simulink model "uvms_sliding_quaternions"  (Simulink 7.9)
settings: Solver=ode4  StartTime=0.0  StopTime=10  FixedStep=dt  RelTol=2*1e-3
values from neighbouring files (symbols this model uses):
  DH = struct('a',zeros(n,1),'d',zeros(n,1),'alpha',zeros(n,1))    [init.m]
  dt = read_config('dt', 'number')    [run_simulation.m]
undefined symbols (not defined in the file or in its folder): commanded_zeta, ee_pose_init, ee_pose_quaternion_init, Kinetics_Parameters, q_init, V_current, vehicle_position_init, vehicle_quaternion_init
libraries: simulink x1
(part 2 of 2)

== matlab function Controller/sliding mode 2/tau1 ==
  data: Kinetics_Parameters input Bus: kinetics_bus; tau output double; Measured_States input Bus: measured_states_bus; Commanded_States input Bus: commanded_states_bus; zetas input double; dzetas input double
function tau = slidingMode(Kinetics_Parameters, Measured_States,Commanded_States, zetas, dzetas)
%#codegen
    
    
    zeta = Measured_States.zeta;
    zetar_est = zeta;
    s = zeta - zetas;
    Mest = 0.9*getM(Measured_States, Kinetics_Parameters);
    Cest = 1.2*getC(Measured_States, Kinetics_Parameters, zeta, zetar_est);
    Dest = 1.3*getD(Measured_States, Kinetics_Parameters, zetar_est);
    Nest = 0.75*getN(Measured_States, Kinetics_Parameters);
    Xiest = zeros(12,1);

    Kd=diag([10, 10, 10 ,15, 20, 15, ...
             10, 10, 10, 10, 10, 10])*1.2;
    Ks=diag([50, 50, 50, 60, 80, 60, ...
             10, 10, 10, 10, 10, 10])*1.5;
   
    tau = Mest* dzetas + Cest* zetas + Dest * zetas + Nest + Xiest - Kd* s - Ks*sat( s, 0.3) ;% Ks*sat( s, 0.5);
    
end

%------------------------------------------------------------------------
% saturation function
function vec = sat (x,epsilon)
    vec=zeros(length(x),1);
    for i=1:length(x)
       if x(i) > epsilon
           vec(i)=1;
       elseif x(i) < -epsilon
           vec(i)=-1;
       else
           vec(i)=x(i)/epsilon;
       end
    end
end


%% --------------------------------------------------------------
%  Functions to gather the vectors   
%%---------------------------------------------------------------

function M = getM(Measured_States, Kinetics_Parameters)
    Mrb = getMrb(Measured_States, Kinetics_Parameters);
    Ma = getMa(Measured_States, Kinetics_Parameters);
    M = (Mrb + Ma);
end


function C = getC (Measured_States,Kinetics_Parameters, zeta ,zetar)
    Crb = getCrb(Measured_States,Kinetics_Parameters, zeta) ;
   	Ca = getCa(Measured_States,Kinetics_Parameters,zetar);
    C = Crb + Ca;
end


%% --------------------------------------------------------------
%  Inertia function   
%%---------------------------------------------------------------
function M = getMrb(Measured_States, Kinetics_Parameters)
%#codegen
%   getMrb Returns the sum of the Rigid body inertia and the added mass:
%   M_rb + M_a
%   
    n=6;
    i=1;
    M = zeros(12,12);
    Inertia = Kinetics_Parameters.Inertia;
    Jgb = [eye(6), zeros(6,6)];                                 % Jacobian from vehicle 
    Ji=Jgb;
    Hi = Kinetics_Parameters.Persistent.Hrg(:,:,i);
    Ii=Hi'*(Inertia(:,:,1))*Hi;                                 % Inertia of vehicle in CO
    M=M+(Ji')*Ii*Ji;
    for i=1:n
        Ji = Measured_States.Ji.Ji(:,:,i);                      % body jacobian
        Hi =Kinetics_Parameters.Persistent.Hrg(:,:,i+1);        % get Transformation matrix of link i
        Ii=Hi'*(Inertia(:,:,i+1) )*Hi;                          % Transform Inertia matrix from CG to CO
        M=M+(Ji')*Ii*Ji;                                        % Add link i's inertia to total inertia
    end
end







%% ------------------------------------------------------
% Persistent Forces   
%%-------------------------------------------------------
function N_p = getN(Measured_States,Kinetics_Parameters)
%#codegen
%   N_p - 12 x 1 vector of generalized forces
%   Persistent_Forces returns the generalized forces due to boyancy and 
%   gravity

    %% init
    n=6;
    
    N_p=zeros(12,1);
    Jgis = Measured_States.Ji.Ji;
    
    %%  vehicle
    F_bp = getFbp(Measured_States, Kinetics_Parameters,1);      % Get wrench from persistent forces in CO
    Jbb=([eye(6), zeros(6,6)]);                                 % Jacobian from b to b
    N_p = Jbb'*F_bp;                                            % Get contribution to total forces through Jbb
    
    %% robot links
    for i=1:n
        Jgi=Jgis(:,:,i);                                        % Jacobian from b to i
        F_ip = getFip(Measured_States,Kinetics_Parameters, i+1);     % Get wrench in CO
        N_p = N_p + (Jgi')*F_ip;                                % Map to generalized forces and add to total
    end
    N_p = - N_p;                                                % reverse the sign to comply with the sign convention
end
    
    
function F_ip = getFip(Measured_States,Kinetics_Parameters, i)
%#codegen
% function calculating wrench from persistent forces 
% i=b: vehicle
% i>=1: robot arms
    F_ip = zeros(6,1);
    mi = Kinetics_Parameters.Persistent.m(i);
    g = Kinetics_Parameters.Persistent.g;
    rho = Kinetics_Parameters.Persistent.rho;
    nabla = Kinetics_Parameters.Persistent.nabla(i);
    Ri0 = Measured_States.Ti.R0i(:,:,i-1)';
    Hrg = Kinetics_Parameters.Persistent.Hrg(:,:,i);  
    Hrb = Kinetics_Parameters.Persistent.Hrb(:,:,i);
    ez=[0;0;1];
    F_ip(:,:) = (Hrg')*[-mi*g*Ri0*ez ;0;0;0]  + (Hrb')*[rho*nabla*g*Ri0*ez ;0;0;0 ];
end


function F_bp = getFbp(Measured_States,Kinetics_Parameters, i)
%#codegen
% function calculating wrench from persistent forces 
% i=b: vehicle
% i>=1: robot arms
    F_bp = zeros(6,1);
    mi = Kinetics_Parameters.Persistent.m(i);
    g = Kinetics_Parameters.Persistent.g;
    Hrg = Kinetics_Parameters.Persistent.Hrg(:,:,i);  
    Hrb = Kinetics_Parameters.Persistent.Hrb(:,:,i);
    rho = Kinetics_Parameters.Persistent.rho;
    nabla = Kinetics_Parameters.Persistent.nabla(i);
    Ri0 = (Measured_States.Ti.R0b)';
    ez=[0;0;1];
    F_bp(:,:) = (Hrg')*[-mi*g*Ri0*ez ; 0;0;0]  + (Hrb')*[rho*nabla*g*Ri0*ez ; 0;0;0 ];
end


%% ------------------------------------------------------
% Coriolis Matrix   
%%-------------------------------------------------------

function C = getCrb(Measured_States,Kinetics_Parameters, zeta)
%#codegen
%-----------------------------------------------------------------------
%   This function calculates the coriolis according to From and Pettersen
%   (2013).
%-----------------------------------------------------------------------
    n=6;
    C=zeros(12,12);
    Inertia=Kinetics_Parameters.Inertia;
    Jis = Measured_States.Ji.Ji;
    
    % i = b
    Jgb = [eye(6), zeros(6,6)];
    i=1;
    Hi = Kinetics_Parameters.Persistent.Hrg(:,:,i);
    Ii=Hi'*Inertia(:,:,i);
    Wb = getWb(Ii,zeta);
    C = - (Jgb')*Wb*Hi*Jgb;     % time derivative of Jgb = 0  
    
    % i >=1
    for i=1:n
        Hi = Kinetics_Parameters.Persistent.Hrg(:,:,i+1);
        Ii=Hi'*Inertia(:,:,i+1);
        Wi=getWi(Ii,Jis(:,:,i), zeta);
        Jgi_dot=getJgi_dot(Measured_States, zeta,i);
        Jgi = Jis(:,:,i);
        
        C = C + (Jgi')*Ii*Hi*Jgi_dot - (Jgi')*Wi*Hi*Jgi;
    end
end



function Wb = getWb(I , zeta)
%#codegen
% Get the matrix Wi for i=b
% I: Inertia matrix for vehicle
% zeta: generalized velocity
    Wb = zeros(6,6);
    v = zeta(1:3);
    omega = zeta(4:6);
    mI = I(1:3,1:3); % Identity matrix times mass of link b
    Ib = I(4:6,4:6); % Moment of inertia
    mrgb = I(4:6,1:3); % mass times skew symmetric r_g^b
    dKv= mI*v - mrgb*omega;
    dKomega = Ib*omega + mrgb*v;
    
    Wb = [zeros(3,3), skew(dKv) ; skew(dKv), skew(dKomega)];
end

function Wi = getWi(I, Ji,zeta)
%#codegen
% Get matrix Wi for robot links
% I: inertia matrix for link i
% Ji: Jacobian for link i
% zeta: generalized coordinates
    Wi = zeros(6,6);
    V0i = Ji*zeta;
    v = V0i(1:3);
    omega = V0i(4:6);
    mI = I(1:3,1:3); % Identity matrix times mass of link b
    Ib = I(4:6,4:6); % Moment of inertia
    mrgb = I(4:6,1:3); % mass times skew symmetric r_g^b
    dKv= mI*v - mrgb*omega;
    dKomega = Ib*omega + mrgb*v;
    Wi = [zeros(3,3), skew(dKv) ; skew(dKv), skew(dKomega)];
end

function Jgi_dot=getJgi_dot(Measured_States, zeta,i)
%#codegen
% the functions below is related to Jgi_dot
    Jgi_dot = zeros(6,6+6);
    n=6;
    Jgi = Measured_States.Ji.Ji(:,:,i);
    omega = Jgi*zeta;
    Rbi = Measured_States.Ti.Rbi(:,:,i);
    pbi = Measured_States.Ti.pbi(:,i);
    omegaib = getOmegaib(Measured_States,zeta,i);
    dpbi =  getDpbi(Measured_States,zeta,i);
        
    dAdg_inv = [(Rbi')*skew(omegaib) , -(Rbi')*skew(omegaib)*skew(pbi) + (Rbi')*skew(dpbi); ...
                zeros(3,3) , (Rbi')*skew(omegaib) ];
    dJi = zeros(6,6);
    omega0b = zeta(4:6);
    
    % get d/dt(Ji)
    Xii=[0,0,0,0,0,1]';
    for k=2:n
       if k<=i
            dpbk = getDpbi(Measured_States, zeta ,k-1);
            Rbk= Measured_States.Ti.Rbi(:,:,k-1);
            omega0k = [zeros(3,3) , eye(3)]*Measured_States.Ji.Ji(:,:,k-1)*zeta;
            omegabk = omega0k - (Rbk')*omega0b;
            dJi(:,k) = [zeros(3,3), skew(dpbk)*Rbk*skew(omegabk) ...
                ; zeros(3,3) , (Rbk')*skew(omegabk)]*Xii;
       end
    end
    Ji=getji(Measured_States.Ti, i);
    Adg_inv = Measured_States.Ti.Adgbi_inv(:,:,i);
    Jgi_dot = [dAdg_inv, dAdg_inv*Ji + Adg_inv*dJi ];
end

function omegaib = getOmegaib(Measured_States,zeta,i)
%#codegen
% returns angular rate of vehcile wrt frame i noted in vehicle frame
    omegaib = zeros(3,1);
    Rbi = Measured_States.Ti.Rbi(:,:,i);
    Jgi = Measured_States.Ji.Ji(:,:,i);
    omega0b = zeta(4:6);
    omegaib = omega0b - Rbi*[zeros(3,3), eye(3)]*Jgi*zeta;
end

function dpbi = getDpbi( Measured_States, zeta,iter)
%#codegen
% returns time derivative of position vector of from frame b to frame i
    dpbi = zeros(3,1);
    H = [eye(3), zeros(3,3)];
    Rbi=Measured_States.Ti.Rbi(:,:,iter);
    Adgbi_inv = Measured_States.Ti.Adgbi_inv(:,:,iter);
    Ji = getji(Measured_States.Ti,iter);
    qd=zeros(6,1);
    qd(:,:)=zeta(7:12);
    dpbi = Rbi*H*Adgbi_inv*Ji*qd;
end


function mat = getji(Ti,i)
%#codegen
% return matrix Ji (see report)
    n=6;
    mat=zeros(6,6);
    Xii=[0,0,0,0,0,1]';
    mat(:,1)=eye(6)*Xii;
    for j=2:n
        if j<=i
            mat(:,j) = Ti.Adgbi(:,:,j-1)*Xii;
        end
    end
end

function S = skew(v)
%#codegen

  S = [  0   -v(3)  v(2)
       v(3)  0    -v(1)
       -v(2) v(1)   0];
end


%% ------------------------------------------------------
% D matrix 
%%-------------------------------------------------------
function D = getD(Measured_States, Kinetics_Parameters,zetar)
%#codegen
%
% Returns the D matrix in the dynamics equation. The total forces is based
% on mappin the forces in each frame to the total generalized forces
% through the jacoian: tau = J^T*F_i. The forces in frame i is calculated
% from the forces in CG to CO through the transformation matrix: F_co =
% Hrg^T*F_cg
%
    %% init
    n=6;
    D=zeros(12,12);                                      % init matrix size
    HydroDynamics = Kinetics_Parameters.HydroDynamics;   % Hydrodynamics parameters
    Jgis = Measured_States.Ji.Ji;                             % Jacobians
    Hrgs = Kinetics_Parameters.Persistent.Hrg;           % Transformation matrix
    
    
    %% vehicle
    i=1;
    Jbb=[eye(6), zeros(6)];                               % Jacobian from frame 0 to frame b
    Hrg = Hrgs(:,:,i);                                    % Transformation matrix
    Vcg = Hrg*Jbb*zetar;                                   % velocity in CG mapped from CO
    Dcg =  HydroDynamics.Linear(:,:,i) + ...
           HydroDynamics.Quadratic(:,:,i)*diag(abs(Vcg)); % Wrench in CG
    Di = Hrg'*Dcg;                                        % Wrench in CO mapped from CG    
    D = Jbb'*Di*Jbb;                                      % Add contribution to the total matrix mapped from frame i 
                                                          % to generalized coordinates                                   
    
    %% robot links
    for i=1:n
        Jgi = Jgis(:,:,i);                                % Jacobian from frame 0 to frame i 
        Hrg = Hrgs(:,:,i+1);                              % Transformation matrix
        Vcg = Hrg*Jgi*zetar;                               % velocity in CG
        Dcg = HydroDynamics.Linear(:,:,i+1)+... 
          HydroDynamics.Quadratic(:,:,i+1)*diag(abs(Vcg));% Wrench in CG   
        Di = Hrg'*Dcg;                                    % Wrench in CO    
        D = D + Jgi'*Di*Jgi;                              % Add frame i's contribution to D matrix    
    end
end

%% ------------------------------------------------------
% Added Coriolis
%%-------------------------------------------------------
function Ca = getCa(Measured_States,Kinetics_Parameters,zetar)
%%#codegen ..............................................
%
%   This function calculates the added coriolis matrix
%.......................................................
    n=6;
    Ca=zeros(12,12);
    Inertia=Kinetics_Parameters.AddedInertia;
    Jis = Measured_States.Ji.Ji;
    
    % vehicle
    Jgb = [eye(6), zeros(6,6)];
    i=1;
    Hi = Kinetics_Parameters.Persistent.Hrg(:,:,i+1);
    Ii=Hi'*Inertia(:,:,i);
    Wb = getWb(Ii,zetar);
    Ca = - (Jgb')*Wb*Hi*Jgb;     % time derivative of Jgb = 0  
    
    % manipulator links
    for i=1:n
        Hi = Kinetics_Parameters.Persistent.Hrg(:,:,i+1);
        Ii=Hi'*Inertia(:,:,i+1);
        Wi=getWi(Ii,Jis(:,:,i), zetar);
        Jgi_dot=getJgi_dot(Measured_States, zetar,i);
        Jgi = Jis(:,:,i);
        Ca = Ca + (Jgi')*Ii*Hi*Jgi_dot - (Jgi')*Wi*Hi*Jgi;
    end
end

%% ------------------------------------------------------
% Added Mass
%%-------------------------------------------------------
function Ma = getMa(Measured_States,Kinetics_Parameters)
%#codegen ..........................
%
%  returns rest of the the added mass
%  force matrix:
%       Ma*H(xi,zeta)
% ..................................
    n=6;
    i=1;
    
    %% get the total Added mass matrix
    Ma = zeros(12,12);
    AddedInertia = Kinetics_Parameters.AddedInertia;
    Jgb = [eye(6), zeros(6,6)];                                 % Jacobian from vehicle 
    Ji=Jgb;
    Hi = Kinetics_Parameters.Persistent.Hrg(:,:,i);
    Ii=Hi'*( AddedInertia(:,:,1))*Hi;                           % Inertia of vehicle in CO
    Ma=Ma+(Ji')*Ii*Ji;
    for i=1:n
        Ji = Measured_States.Ji.Ji(:,:,i);                           % body jacobian
        Hi =Kinetics_Parameters.Persistent.Hrg(:,:,i+1);        % get Transformation matrix of link i
        Ii=Hi'*(AddedInertia(:,:,i+1))*Hi;                      % Transform Inertia matrix from CG to CO
        Ma=Ma+(Ji')*Ii*Ji;                                      % Add link i's inertia to total inertia
    end
 end

== matlab function UVMS/End Effector2/twist2pose_quaternions/MATLAB Function ==
  data: pose output double; quaternion output double; poseIn input double
function [pose, quaternion] = fcn(poseIn)
%#codegen
    pose = poseIn;
    quaternion = poseIn(4:7);
end

== matlab function UVMS/End Effector2/twist2pose_quaternions/body2quat ==
  data: ee_velocity_twist input double size=6; ee_rates output double; quat input double
function ee_rates = fcn(ee_velocity_twist, quat)                       
    %#codegen
    
    eta  = quat(1); 
    eps1 = quat(2); 
    eps2 = quat(3); 
    eps3 = quat(4); 
    
    
    normalization_feedback = getNormalizationFeedback(quat);
    
    v = ee_velocity_twist(1:3);
    omega = ee_velocity_twist(4:6);
    
    R = Rquat(quat);

    T = 0.5*[...
    -eps1 -eps2 -eps3        
    eta  -eps3  eps2
    eps3  eta  -eps1
    -eps2  eps1  eta   ];

    pdot = R*v;
    qdot = T*omega + normalization_feedback;
    
    ee_rates = zeros(7,1);
    ee_rates(:) = [pdot;    0*  qdot];
    
end



function R = Rquat(q)
%#codegen
eta = q(1);
eps = q(2:4);
S = skew(eps);
R = eye(3) + 2*eta*S + 2*S^2;

end


function S = skew(v)
%#codegen
    S = [  0   -v(3)  v(2)
       v(3)  0    -v(1)
       -v(2) v(1)   0];
end


%----------------------------------------------------------------
%   use normalization feedback according to fossen
%   page 31
%
function qout = getNormalizationFeedback(qin)
%#codegen
    qout = zeros(4,1);
    gamma = 100;
    qout = gamma*0.5*(1-qin'*qin)*qin;

end
